simulink model "simulateFlight"  (R2024b)
settings: Solver=VariableStepAuto  StartTime=0.0  StopTime=10
undefined symbols (not defined in the file): aerodynamicData, aircraftConfiguration, alpha0, inertialData, propulsionData, q0, theta0, V0, xE0, zE0
libraries: simulink_extras x8, aerolibatmos2 x2, aerolibanim x1, simulink x1
settings Model: NumberOfSteps=10  VariantFading=off  Creator=vince  LastModifiedBy=klakhara
settings SolverCC: ZeroCrossAlgorithm=Adaptive
settings DebuggingCC: AlgebraicLoopMsg=none  IgnoredZcDiagnostic=none
settings RTWCC: GPUComputeCapability=3.5

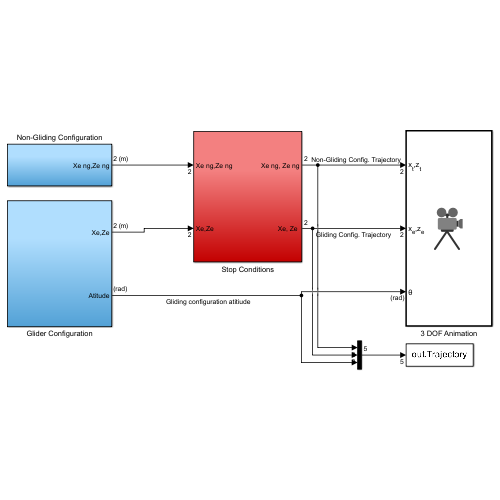
[thumbnail: Simulink's stored preview of the top-level diagram]
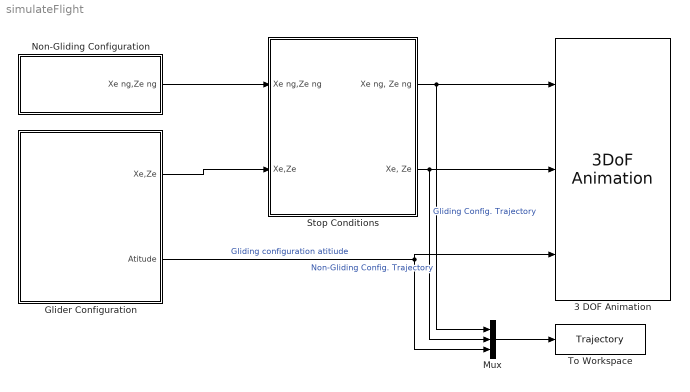
== system simulateFlight ==
  3 DOF Animation : aerolibanim/3DoF Animation  u1=[0 100 0 100 -100 0]  u2=0.01  u3=0.15  u5=Fixed position  u6=[0 50 -0]  u7=40  u8=on
  Glider Configuration : Subsystem
  Mux : Mux  Inputs=3
  Non-Gliding Configuration : Subsystem
  Stop Conditions : Subsystem
  To Workspace : ToWorkspace  VariableName=Trajectory  SaveFormat=Timeseries  SampleTime=-1
  wires:
  Non-Gliding Configuration/1(Xe ng,Ze ng) -> Stop Conditions/1(Xe ng,Ze ng)
  Stop Conditions/1("Xe ng, Ze ng") -> Mux/1, 3 DOF Animation/1  "Non-Gliding Config. Trajectory"
  Glider Configuration/2(Atitude) -> 3 DOF Animation/3, Mux/3  "Gliding configuration atitiude"
  Glider Configuration/1(Xe,Ze) -> Stop Conditions/2(Xe,Ze)
  Stop Conditions/2("Xe, Ze ") -> Mux/2, 3 DOF Animation/2  "Gliding Config. Trajectory"
  Mux/1 -> To Workspace/1

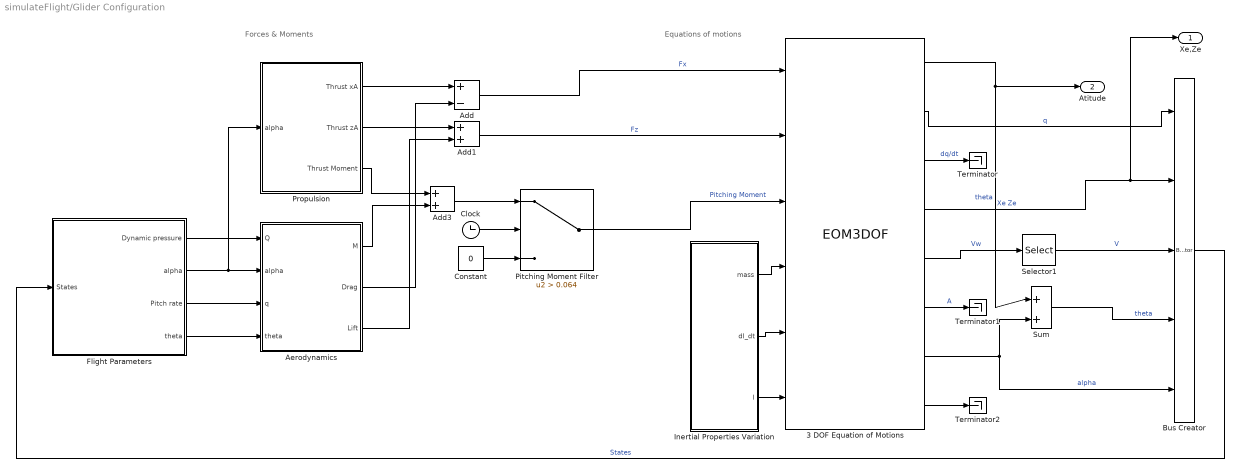
== system simulateFlight/Glider Configuration ==
  note: Forces & Moments
  note: Equations of motions
  3 DOF Equation of Motions : EOM3DOF  axes=Wind  mtype=Custom Variable  v_ini=V0  theta_ini=theta0  gamma_ini=theta0-alpha0  q_ini=q0  alpha_ini=alpha0  pos_ini=[xE0 -zE0]  mass=1  Iyy=1  abi_flag=on
  Add : Sum  Inputs=+-
  Add1 : Sum
  Add3 : Sum
  Aerodynamics : Subsystem
  Bus Creator : BusCreator  Inputs=5
  Clock : Clock
  Constant : Constant  Value=0
  Flight Parameters : Subsystem
  Inertial Properties Variation : Subsystem
  Pitching Moment Filter : Switch  Criteria=u2 > Threshold  Threshold=0.064  SaturateOnIntegerOverflow=off  InputSameDT=off
  Propulsion : Subsystem
  Selector1 : Selector  InputPortWidth=2  IndexOptions=Index vector (dialog)  Indices=[1]  OutputSizes=1
  Sum : Sum  Inputs=|++
  Terminator : Terminator
  Terminator1 : Terminator
  Terminator2 : Terminator
  Xe,Ze : Outport  InitialOutput=0  VectorParamsAs1DForOutWhenUnconnected=off
  Atitude : Outport  Port=2
  wires:
  3 DOF Equation of Motions/5 -> Selector1/1  "Vw"
  Inertial Properties Variation/3(I) -> 3 DOF Equation of Motions/6
  3 DOF Equation of Motions/2 -> Bus Creator/1  "q"
  Pitching Moment Filter/1 -> 3 DOF Equation of Motions/3  "Pitching Moment"
  Inertial Properties Variation/1(mass) -> 3 DOF Equation of Motions/4
  Inertial Properties Variation/2(dI_dt) -> 3 DOF Equation of Motions/5
  3 DOF Equation of Motions/3 -> Terminator/1  "dq/dt"
  3 DOF Equation of Motions/6 -> Terminator1/1  "A"
  Propulsion/3(Thrust Moment) -> Add3/1
  Aerodynamics/1(" M") -> Add3/2
  Aerodynamics/3(Lift) -> Add1/2
  Propulsion/1(Thrust xA) -> Add/1
  Propulsion/2(Thrust zA) -> Add1/1
  Aerodynamics/2(Drag) -> Add/2
  Add1/1 -> 3 DOF Equation of Motions/2  "Fz"
  Add/1 -> 3 DOF Equation of Motions/1  "Fx"
  Add3/1 -> Pitching Moment Filter/1
  3 DOF Equation of Motions/8 -> Terminator2/1
  3 DOF Equation of Motions/7 -> Sum/2, Bus Creator/5  "alpha"
  Selector1/1 -> Bus Creator/3  "V"
  3 DOF Equation of Motions/4 -> Xe,Ze/1, Bus Creator/2  "Xe Ze"
  3 DOF Equation of Motions/1 -> Sum/1, Atitude/1  "theta"
  Flight Parameters/2(alpha) -> Propulsion/1(alpha), Aerodynamics/2(alpha)
  Bus Creator/1 -> Flight Parameters/1(States)  "States"
  Clock/1 -> Pitching Moment Filter/2
  Constant/1 -> Pitching Moment Filter/3
  Flight Parameters/3(Pitch rate) -> Aerodynamics/3(q)
  Flight Parameters/4(theta) -> Aerodynamics/4(theta)
  Flight Parameters/1(Dynamic pressure) -> Aerodynamics/1(Q)
  Sum/1 -> Bus Creator/4  "theta"

== system simulateFlight/Non-Gliding Configuration ==
  Aerodynamics & Equations of Motion : Subsystem
  Dynamic pressure Computation : Subsystem
  Hold : Subsystem
  Thrust Profile : Subsystem
  Xe ng,Ze ng : Outport  InitialOutput=0  VectorParamsAs1DForOutWhenUnconnected=off
  wires:
  Dynamic pressure Computation/1(Q) -> Aerodynamics & Equations of Motion/1(Q)
  Aerodynamics & Equations of Motion/5(Attitude) -> Hold/5(theta)
  Thrust Profile/1(Thrust) -> Aerodynamics & Equations of Motion/5(Thrust)
  Aerodynamics & Equations of Motion/1(V(wind)) -> Hold/1("V(wind) ")
  Aerodynamics & Equations of Motion/2(alpha new) -> Hold/2(alpha)
  Aerodynamics & Equations of Motion/3(q new) -> Hold/3("q ")
  Hold/4(q hold) -> Aerodynamics & Equations of Motion/3(q)
  Hold/1(Xe,Ze hold) -> Dynamic pressure Computation/1("Xe, Ze")
  Hold/2(V(wind) hold) -> Dynamic pressure Computation/2(V(wind))
  Hold/3(alpha hold) -> Aerodynamics & Equations of Motion/2(alpha)
  Hold/5(theta hold) -> Aerodynamics & Equations of Motion/4(theta)
  Aerodynamics & Equations of Motion/4(Xe,Ze) -> Hold/4(Xe,Ze), Xe ng,Ze ng/1

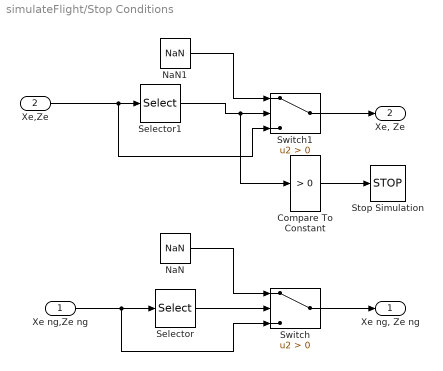
== system simulateFlight/Stop Conditions ==
  Xe ng,Ze ng : Inport
  Xe,Ze : Inport  Port=2
  Compare To Constant : simulink/Logic and Bit Operations/Compare To Constant  relop=>  const=0  OutDataTypeStr=boolean
  NaN : Constant  Value=NaN  OutDataTypeStr=Inherit: Inherit via back propagation
  NaN1 : Constant  Value=NaN  OutDataTypeStr=Inherit: Inherit via back propagation
  Selector : Selector  InputPortWidth=2  IndexOptions=Index vector (dialog)  Indices=[2]  OutputSizes=1
  Selector1 : Selector  InputPortWidth=2  IndexOptions=Index vector (dialog)  Indices=[2]  OutputSizes=1
  Stop Simulation : Stop
  Switch : Switch  Criteria=u2 > Threshold  SaturateOnIntegerOverflow=off  InputSameDT=off
  Switch1 : Switch  Criteria=u2 > Threshold  SaturateOnIntegerOverflow=off  InputSameDT=off
  "Xe ng, Ze ng" : Outport
  "Xe, Ze " : Outport  Port=2
  wires:
  Compare To Constant/1 -> Stop Simulation/1
  Selector/1 -> Switch/2
  NaN/1 -> Switch/1
  Switch/1 -> "Xe ng, Ze ng"/1
  Xe ng,Ze ng/1 -> Switch/3, Selector/1
  Xe,Ze/1 -> Switch1/3, Selector1/1
  Selector1/1 -> Compare To Constant/1, Switch1/2
  NaN1/1 -> Switch1/1
  Switch1/1 -> "Xe, Ze "/1

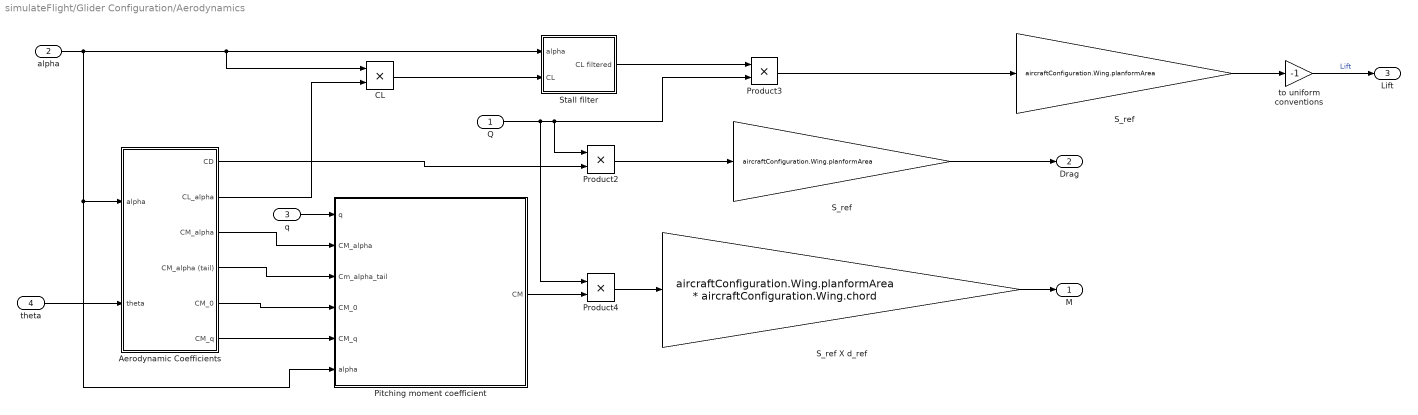
== system simulateFlight/Glider Configuration/Aerodynamics ==
  Q : Inport
  alpha : Inport  Port=2
  q : Inport  Port=3
  theta : Inport  Port=4
  Aerodynamic Coefficients : Subsystem
  CL : Product
  Pitching moment coefficient : Subsystem
  Product2 : Product  InputSameDT=on  SaturateOnIntegerOverflow=on  OutDataTypeStr=Inherit: Same as first input
  Product3 : Product  InputSameDT=on  SaturateOnIntegerOverflow=on  OutDataTypeStr=Inherit: Same as first input
  Product4 : Product  InputSameDT=on  SaturateOnIntegerOverflow=on  OutDataTypeStr=Inherit: Same as first input
  S_ref : Gain  Gain=aircraftConfiguration.Wing.planformArea  SaturateOnIntegerOverflow=on  OutDataTypeStr=Inherit: Same as input  ParamDataTypeStr=Inherit: Same as input
  "S_ref " : Gain  Gain=aircraftConfiguration.Wing.planformArea  SaturateOnIntegerOverflow=on  OutDataTypeStr=Inherit: Same as input  ParamDataTypeStr=Inherit: Same as input
  S_ref X d_ref : Gain  Gain=aircraftConfiguration.Wing.planformArea * aircraftConfiguration.Wing.chord  SaturateOnIntegerOverflow=on  OutDataTypeStr=Inherit: Same as input  ParamDataTypeStr=Inherit: Same as input
  Stall filter : Subsystem
  to uniform conventions : Gain  Gain=-1
  " M" : Outport  InitialOutput=0  VectorParamsAs1DForOutWhenUnconnected=off
  Drag : Outport  Port=2  InitialOutput=[0]  VectorParamsAs1DForOutWhenUnconnected=off
  Lift : Outport  Port=3  InitialOutput=0  VectorParamsAs1DForOutWhenUnconnected=off
  wires:
  theta/1 -> Aerodynamic Coefficients/2(theta)
  alpha/1 -> Stall filter/1(alpha), CL/1, Pitching moment coefficient/6(alpha), Aerodynamic Coefficients/1(alpha)
  S_ref X d_ref/1 -> " M"/1
  q/1 -> Pitching moment coefficient/1(q)
  Aerodynamic Coefficients/2(CL_alpha) -> CL/2
  Aerodynamic Coefficients/1(CD) -> Product2/2
  Aerodynamic Coefficients/3(CM_alpha) -> Pitching moment coefficient/2(CM_alpha)
  Aerodynamic Coefficients/4(CM_alpha (tail)) -> Pitching moment coefficient/3(Cm_alpha_tail)
  Aerodynamic Coefficients/5(CM_0) -> Pitching moment coefficient/4(CM_0)
  Aerodynamic Coefficients/6(CM_q) -> Pitching moment coefficient/5(CM_q)
  CL/1 -> Stall filter/2(CL)
  Q/1 -> Product3/2, Product2/1, Product4/1
  "S_ref "/1 -> to uniform conventions/1
  Pitching moment coefficient/1(CM) -> Product4/2
  Stall filter/1(CL filtered) -> Product3/1
  Product2/1 -> S_ref/1
  Product4/1 -> S_ref X d_ref/1
  Product3/1 -> "S_ref "/1
  S_ref/1 -> Drag/1
  to uniform conventions/1 -> Lift/1  "Lift"

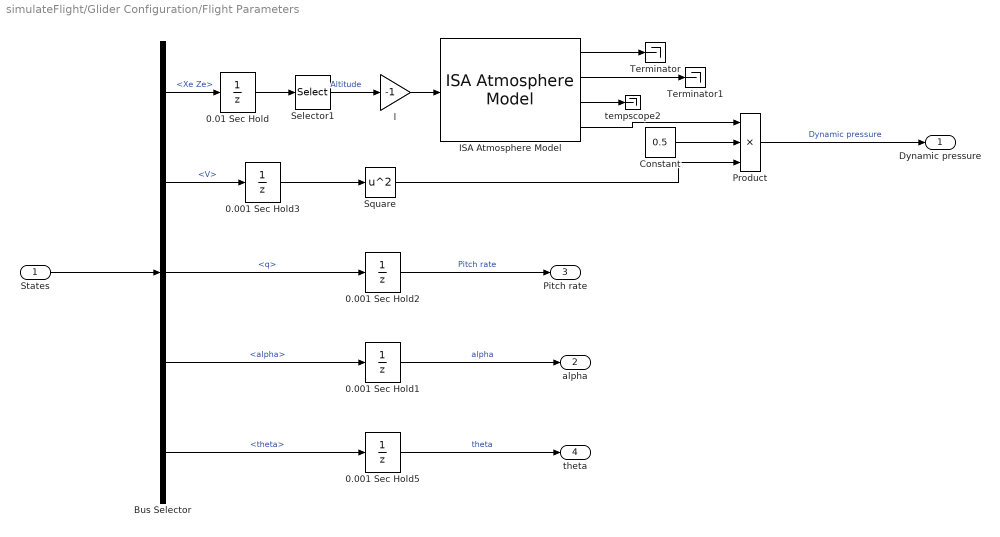
== system simulateFlight/Glider Configuration/Flight Parameters ==
  States : Inport
  0.001 Sec Hold1 : UnitDelay  InitialCondition=alpha0  SampleTime=0.001  HasFrameUpgradeWarning=on
  0.001 Sec Hold2 : UnitDelay  InitialCondition=q0  SampleTime=0.001  HasFrameUpgradeWarning=on
  0.001 Sec Hold3 : UnitDelay  InitialCondition=V0  SampleTime=0.001  HasFrameUpgradeWarning=on
  0.001 Sec Hold5 : UnitDelay  InitialCondition=theta0  SampleTime=0.001  HasFrameUpgradeWarning=on
  0.01 Sec Hold : UnitDelay  InitialCondition=[xE0 -zE0]  SampleTime=0.01  HasFrameUpgradeWarning=on
  Bus Selector : BusSelector  OutputSignals=Xe Ze,V,q,alpha,theta
  Constant : Constant  Value=0.5
  ISA Atmosphere Model : aerolibatmos2/ISA Atmosphere Model  useExtended=off  action=Warning  custom=off  viscosityOut=off  g=9.80665  gamma=1.4  R=287.0531  L=0.0065  h_trop=11000  h_strat=20000  rho0=1.225  P0=101325  T0=288.15  h0=0  S=110.4  Tref=273.15  muref=1.716e-5
  Product : Product  Inputs=3
  Selector1 : Selector  InputPortWidth=2  IndexOptions=Index vector (dialog)  Indices=[2]  OutputSizes=1
  Square : Math  Operator=square
  Terminator : Terminator
  Terminator1 : Terminator
  l : Gain  Gain=-1  SaturateOnIntegerOverflow=on  OutDataTypeStr=Inherit: Same as input  ParamDataTypeStr=Inherit: Same as input
  tempscope2 : Terminator
  Dynamic pressure : Outport
  alpha : Outport  Port=2
  Pitch rate : Outport  Port=3
  theta : Outport  Port=4
  wires:
  Bus Selector/3 -> 0.001 Sec Hold2/1  "<q>"
  Bus Selector/1 -> 0.01 Sec Hold/1  "<Xe Ze>"
  ISA Atmosphere Model/2 -> Terminator1/1
  ISA Atmosphere Model/4 -> Product/1
  0.001 Sec Hold3/1 -> Square/1
  ISA Atmosphere Model/3 -> tempscope2/1
  Bus Selector/2 -> 0.001 Sec Hold3/1  "<V>"
  Bus Selector/4 -> 0.001 Sec Hold1/1  "<alpha>"
  l/1 -> ISA Atmosphere Model/1
  0.001 Sec Hold2/1 -> Pitch rate/1  "Pitch rate"
  Selector1/1 -> l/1  "Altitude"
  0.01 Sec Hold/1 -> Selector1/1
  Bus Selector/5 -> 0.001 Sec Hold5/1  "<theta>"
  Square/1 -> Product/3
  Product/1 -> Dynamic pressure/1  "Dynamic pressure"
  ISA Atmosphere Model/1 -> Terminator/1
  States/1 -> Bus Selector/1
  0.001 Sec Hold5/1 -> theta/1  "theta"
  0.001 Sec Hold1/1 -> alpha/1  "alpha"
  Constant/1 -> Product/2

== system simulateFlight/Glider Configuration/Inertial Properties Variation ==
  Clock : Clock
  Derivative : Derivative
  Inertia moment vs time : Lookup_n-D  NumberOfTableDimensions=1  BreakpointsForDimension1=inertialData.massTimeRange  Table=inertialData.inertiaVector  InternalRulePriority=Speed  RndMeth=Simplest
  mass vs time : Lookup_n-D  NumberOfTableDimensions=1  BreakpointsForDimension1=inertialData.massTimeRange  Table=inertialData.massVector  ExtrapMethod=Clip  InternalRulePriority=Speed  RndMeth=Simplest
  mass : Outport
  dI_dt : Outport  Port=2
  I : Outport  Port=3
  wires:
  Clock/1 -> mass vs time/1, Inertia moment vs time/1
  mass vs time/1 -> mass/1
  Derivative/1 -> dI_dt/1
  Inertia moment vs time/1 -> I/1, Derivative/1

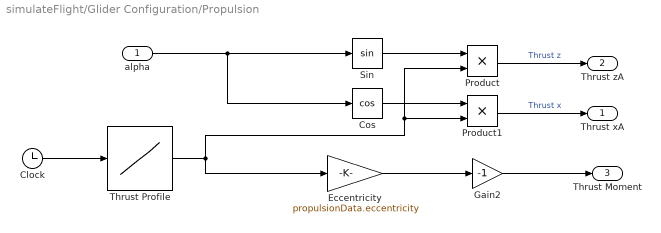
== system simulateFlight/Glider Configuration/Propulsion ==
  alpha : Inport
  Clock : Clock
  Cos : Trigonometry  Operator=cos
  Eccentricity : Gain  Gain=propulsionData.eccentricity
  Gain2 : Gain  Gain=-1
  Product : Product
  Product1 : Product
  Sin : Trigonometry
  Thrust Profile : Lookup_n-D  NumberOfTableDimensions=1  BreakpointsForDimension1=propulsionData.thrustTimeRange  Table=propulsionData.thrustVector  InternalRulePriority=Speed  RndMeth=Simplest
  Thrust xA : Outport
  Thrust zA : Outport  Port=2
  Thrust Moment : Outport  Port=3
  wires:
  alpha/1 -> Cos/1, Sin/1
  Cos/1 -> Product1/1
  Sin/1 -> Product/1
  Product/1 -> Thrust zA/1  "Thrust z"
  Product1/1 -> Thrust xA/1  "Thrust x"
  Thrust Profile/1 -> Eccentricity/1, Product1/2, Product/2
  Eccentricity/1 -> Gain2/1
  Gain2/1 -> Thrust Moment/1
  Clock/1 -> Thrust Profile/1

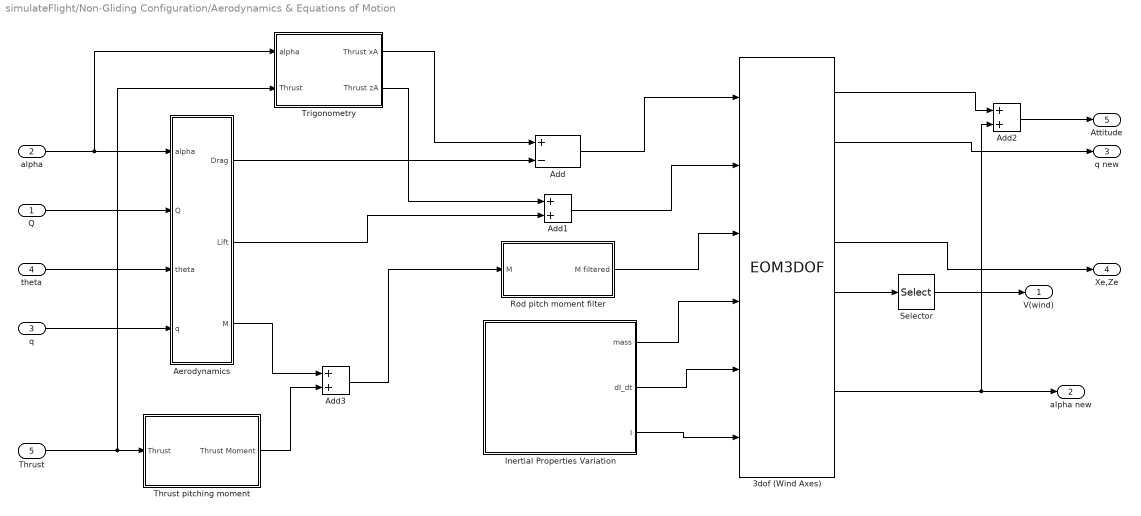
== system simulateFlight/Non-Gliding Configuration/Aerodynamics & Equations of Motion ==
  Q : Inport
  alpha : Inport  Port=2
  q : Inport  Port=3
  theta : Inport  Port=4
  Thrust : Inport  Port=5
  3dof (Wind Axes) : EOM3DOF  axes=Wind  mtype=Custom Variable  v_ini=V0  theta_ini=theta0  gamma_ini=theta0-alpha0  q_ini=q0  alpha_ini=alpha0  pos_ini=[xE0 zE0]  abi_flag=on
  Add : Sum  Inputs=+-
  Add1 : Sum
  Add2 : Sum
  Add3 : Sum
  Aerodynamics : Subsystem
  Inertial Properties Variation : Subsystem
  Rod pitch moment filter : Subsystem
  Selector : Selector  NumberOfDimensions=2  InputPortWidth=3  IndexOptions=Index vector (dialog),Index vector (dialog)  Indices=1,1  OutputSizes=1,1
  Thrust pitching moment : Subsystem
  Trigonometry : Subsystem
  V(wind) : Outport  InitialOutput=0  VectorParamsAs1DForOutWhenUnconnected=off
  alpha new : Outport  Port=2  InitialOutput=0  VectorParamsAs1DForOutWhenUnconnected=off
  q new : Outport  Port=3  InitialOutput=0  VectorParamsAs1DForOutWhenUnconnected=off
  Xe,Ze : Outport  Port=4  InitialOutput=0  VectorParamsAs1DForOutWhenUnconnected=off
  Attitude : Outport  Port=5  InitialOutput=0  VectorParamsAs1DForOutWhenUnconnected=off
  wires:
  Add/1 -> 3dof (Wind Axes)/1
  Q/1 -> Aerodynamics/2(Q)
  3dof (Wind Axes)/4 -> Xe,Ze/1
  3dof (Wind Axes)/1 -> Add2/1
  theta/1 -> Aerodynamics/3(theta)
  alpha/1 -> Aerodynamics/1(alpha), Trigonometry/1(alpha)
  Trigonometry/2(Thrust zA) -> Add1/1
  Aerodynamics/2(Lift) -> Add1/2
  3dof (Wind Axes)/5 -> Selector/1
  Thrust/1 -> Trigonometry/2(Thrust), Thrust pitching moment/1(Thrust)
  3dof (Wind Axes)/2 -> q new/1
  q/1 -> Aerodynamics/4(q)
  Aerodynamics/1(Drag) -> Add/2
  Trigonometry/1(Thrust xA) -> Add/1
  Add1/1 -> 3dof (Wind Axes)/2
  Rod pitch moment filter/1(M filtered) -> 3dof (Wind Axes)/3
  Thrust pitching moment/1(Thrust Moment) -> Add3/2
  Aerodynamics/3(" M") -> Add3/1
  Add3/1 -> Rod pitch moment filter/1(M)
  Inertial Properties Variation/1(mass) -> 3dof (Wind Axes)/4
  Inertial Properties Variation/2(dI_dt) -> 3dof (Wind Axes)/5
  Inertial Properties Variation/3(I) -> 3dof (Wind Axes)/6
  Selector/1 -> V(wind)/1
  3dof (Wind Axes)/7 -> Add2/2, alpha new/1
  Add2/1 -> Attitude/1

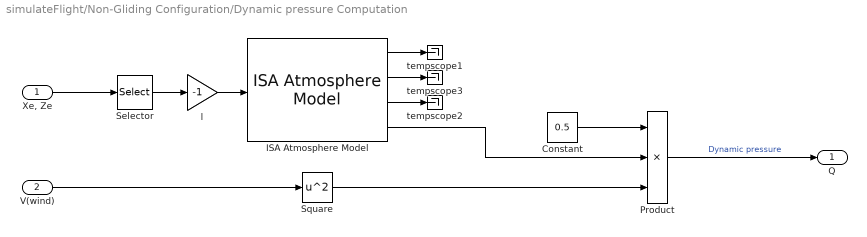
== system simulateFlight/Non-Gliding Configuration/Dynamic pressure Computation ==
  "Xe, Ze" : Inport
  V(wind) : Inport  Port=2
  Constant : Constant  Value=0.5
  ISA Atmosphere Model : aerolibatmos2/ISA Atmosphere Model  useExtended=off  action=Warning  custom=off  viscosityOut=off  g=9.80665  gamma=1.4  R=287.0531  L=0.0065  h_trop=11000  h_strat=20000  rho0=1.225  P0=101325  T0=288.15  h0=0  S=110.4  Tref=273.15  muref=1.716e-5
  Product : Product  Inputs=3
  Selector : Selector  InputPortWidth=2  IndexOptions=Index vector (dialog)  Indices=[2]  OutputSizes=1
  Square : Math  Operator=square
  l : Gain  Gain=-1  SaturateOnIntegerOverflow=on  OutDataTypeStr=Inherit: Same as input  ParamDataTypeStr=Inherit: Same as input
  tempscope1 : Terminator
  tempscope2 : Terminator
  tempscope3 : Terminator
  Q : Outport
  wires:
  l/1 -> ISA Atmosphere Model/1
  ISA Atmosphere Model/1 -> tempscope1/1
  ISA Atmosphere Model/3 -> tempscope2/1
  Selector/1 -> l/1
  Product/1 -> Q/1  "Dynamic pressure"
  Constant/1 -> Product/1
  ISA Atmosphere Model/4 -> Product/2
  Square/1 -> Product/3
  "Xe, Ze"/1 -> Selector/1
  V(wind)/1 -> Square/1
  ISA Atmosphere Model/2 -> tempscope3/1

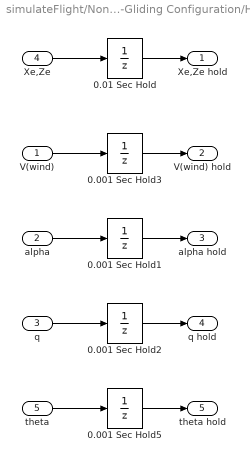
== system simulateFlight/Non-Gliding Configuration/Hold ==
  "V(wind) " : Inport
  alpha : Inport  Port=2
  "q " : Inport  Port=3
  Xe,Ze : Inport  Port=4
  theta : Inport  Port=5
  0.001 Sec Hold1 : UnitDelay  InitialCondition=alpha0  SampleTime=0.001  HasFrameUpgradeWarning=on
  0.001 Sec Hold2 : UnitDelay  InitialCondition=q0  SampleTime=0.001  HasFrameUpgradeWarning=on
  0.001 Sec Hold3 : UnitDelay  InitialCondition=V0  SampleTime=0.001  HasFrameUpgradeWarning=on
  0.001 Sec Hold5 : UnitDelay  InitialCondition=theta0  SampleTime=0.001  HasFrameUpgradeWarning=on
  0.01 Sec Hold : UnitDelay  InitialCondition=[xE0 -zE0]  SampleTime=0.01  HasFrameUpgradeWarning=on
  Xe,Ze hold : Outport
  V(wind) hold : Outport  Port=2
  alpha hold : Outport  Port=3
  q hold : Outport  Port=4
  theta hold : Outport  Port=5
  wires:
  alpha/1 -> 0.001 Sec Hold1/1
  0.001 Sec Hold3/1 -> V(wind) hold/1
  "V(wind) "/1 -> 0.001 Sec Hold3/1
  Xe,Ze/1 -> 0.01 Sec Hold/1
  "q "/1 -> 0.001 Sec Hold2/1
  0.001 Sec Hold2/1 -> q hold/1
  0.01 Sec Hold/1 -> Xe,Ze hold/1
  0.001 Sec Hold1/1 -> alpha hold/1
  theta/1 -> 0.001 Sec Hold5/1
  0.001 Sec Hold5/1 -> theta hold/1

== system simulateFlight/Non-Gliding Configuration/Thrust Profile ==
  1-D Lookup Table : Lookup_n-D  NumberOfTableDimensions=1  BreakpointsForDimension1=propulsionData.thrustTimeRange  Table=propulsionData.thrustVector  InternalRulePriority=Speed  RndMeth=Simplest
  Clock : Clock
  Scope : Scope  NumInputPorts=2
  Thrust : Outport
  wires:
  Clock/1 -> 1-D Lookup Table/1
  1-D Lookup Table/1 -> Scope/1, Thrust/1

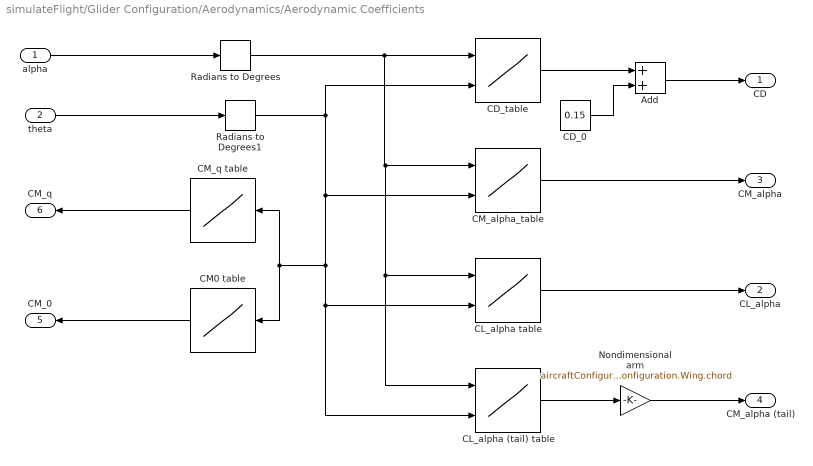
== system simulateFlight/Glider Configuration/Aerodynamics/Aerodynamic Coefficients ==
  alpha : Inport
  theta : Inport  Port=2
  Add : Sum
  CD_0 : Constant  Value=0.15
  CD_table : Lookup_n-D  BreakpointsForDimension1=aerodynamicData.alphaRange  BreakpointsForDimension2=aerodynamicData.thetaRange  Table=aerodynamicData.dragCoefficient.CD_table  ExtrapMethod=Clip  InternalRulePriority=Speed  RndMeth=Simplest
      settings: InputPortMap=u0,u1
  CL_alpha (tail) table : Lookup_n-D  BreakpointsForDimension1=aerodynamicData.alphaRange  BreakpointsForDimension2=aerodynamicData.thetaRange  Table=aerodynamicData.liftCoefficient.CL_alpha_tail_table  InternalRulePriority=Speed  RndMeth=Simplest
      settings: InputPortMap=u0,u1
  CL_alpha table : Lookup_n-D  BreakpointsForDimension1=aerodynamicData.alphaRange  BreakpointsForDimension2=aerodynamicData.thetaRange  Table=aerodynamicData.liftCoefficient.CL_alpha_table  ExtrapMethod=Clip  InternalRulePriority=Speed  RndMeth=Simplest
      settings: InputPortMap=u0,u1
  CM0 table : Lookup_n-D  NumberOfTableDimensions=1  BreakpointsForDimension1=aerodynamicData.thetaRange  Table=aerodynamicData.pitchMomentCoefficient.CM_0  InternalRulePriority=Speed  RndMeth=Simplest
  CM_alpha_table : Lookup_n-D  BreakpointsForDimension1=aerodynamicData.alphaRange  BreakpointsForDimension2=aerodynamicData.thetaRange  Table=aerodynamicData.pitchMomentCoefficient.CM_alpha_table  ExtrapMethod=Clip  InternalRulePriority=Speed  RndMeth=Simplest
      settings: InputPortMap=u0,u1
  CM_q table : Lookup_n-D  NumberOfTableDimensions=1  BreakpointsForDimension1=aerodynamicData.thetaRange  Table=aerodynamicData.pitchMomentCoefficient.Cm_q  InternalRulePriority=Speed  RndMeth=Simplest
  Nondimensional arm : Gain  Gain=aircraftConfiguration.HT.Arm/aircraftConfiguration.Wing.chord
  Radians to Degrees : simulink_extras/Transformations/Radians to Degrees
  Radians to Degrees1 : simulink_extras/Transformations/Radians to Degrees
  CD : Outport
  CL_alpha : Outport  Port=2
  CM_alpha : Outport  Port=3
  CM_alpha (tail) : Outport  Port=4
  CM_0 : Outport  Port=5
  CM_q : Outport  Port=6
  wires:
  alpha/1 -> Radians to Degrees/1
  Radians to Degrees/1 -> CL_alpha (tail) table/1, CL_alpha table/1, CM_alpha_table/1, CD_table/1
  Radians to Degrees1/1 -> CL_alpha (tail) table/2, CL_alpha table/2, CM0 table/1, CM_q table/1, CM_alpha_table/2, CD_table/2
  theta/1 -> Radians to Degrees1/1
  CM_alpha_table/1 -> CM_alpha/1
  CM0 table/1 -> CM_0/1
  Add/1 -> CD/1
  Nondimensional arm/1 -> CM_alpha (tail)/1
  CM_q table/1 -> CM_q/1
  CL_alpha table/1 -> CL_alpha/1
  CL_alpha (tail) table/1 -> Nondimensional arm/1
  CD_table/1 -> Add/1
  CD_0/1 -> Add/2

== system simulateFlight/Glider Configuration/Aerodynamics/Pitching moment coefficient ==
  q : Inport
  CM_alpha : Inport  Port=2
  Cm_alpha_tail : Inport  Port=3
  CM_0 : Inport  Port=4
  CM_q : Inport  Port=5
  alpha : Inport  Port=6
  Add : Sum  Inputs=++++
  CM(a) : Product
  CM(q) : Product
  CM(tail) : Product
  CM_scope : Scope  NumInputPorts=5
  CM : Outport
  wires:
  CM(q)/1 -> Add/4, CM_scope/5
  CM(a)/1 -> Add/2, CM_scope/3
  alpha/1 -> CM(a)/2, CM(tail)/1
  q/1 -> CM(q)/2
  CM(tail)/1 -> Add/3, CM_scope/4
  Add/1 -> CM_scope/1, CM/1  "Resultant"
  CM_q/1 -> CM(q)/1
  CM_alpha/1 -> CM(a)/1
  Cm_alpha_tail/1 -> CM(tail)/2
  CM_0/1 -> Add/1, CM_scope/2

== system simulateFlight/Glider Configuration/Aerodynamics/Stall filter ==
  note: The aircraft stalls at 17 degrees of angle of attack
  alpha : Inport
  CL : Inport  Port=2
  Constant : Constant  Value=0
  Radians to Degrees : simulink_extras/Transformations/Radians to Degrees
  Switch : Switch  Criteria=u2 > Threshold  Threshold=17  SaturateOnIntegerOverflow=off  InputSameDT=off
  CL filtered : Outport
  wires:
  alpha/1 -> Radians to Degrees/1
  Radians to Degrees/1 -> Switch/2
  CL/1 -> Switch/3
  Constant/1 -> Switch/1
  Switch/1 -> CL filtered/1

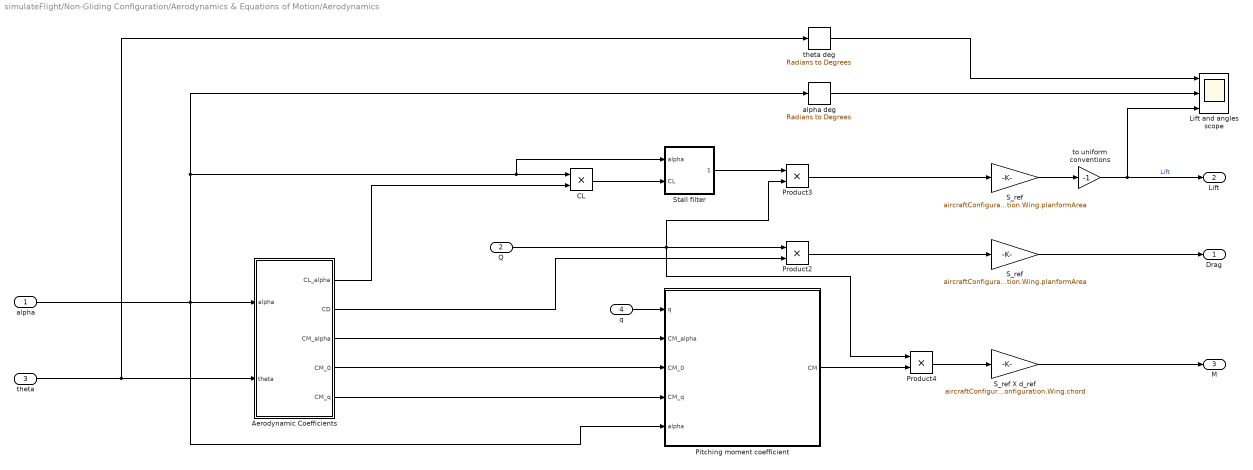
== system simulateFlight/Non-Gliding Configuration/Aerodynamics & Equations of Motion/Aerodynamics ==
  alpha : Inport
  Q : Inport  Port=2
  theta : Inport  Port=3
  q : Inport  Port=4
  Aerodynamic Coefficients : Subsystem
  CL : Product
  Lift and angles scope : Scope  NumInputPorts=3
  Pitching moment coefficient : Subsystem
  Product2 : Product  InputSameDT=on  SaturateOnIntegerOverflow=on  OutDataTypeStr=Inherit: Same as first input
  Product3 : Product  InputSameDT=on  SaturateOnIntegerOverflow=on  OutDataTypeStr=Inherit: Same as first input
  Product4 : Product  InputSameDT=on  SaturateOnIntegerOverflow=on  OutDataTypeStr=Inherit: Same as first input
  S_ref : Gain  Gain=aircraftConfiguration.Wing.planformArea  SaturateOnIntegerOverflow=on  OutDataTypeStr=Inherit: Same as input  ParamDataTypeStr=Inherit: Same as input
  "S_ref " : Gain  Gain=aircraftConfiguration.Wing.planformArea  SaturateOnIntegerOverflow=on  OutDataTypeStr=Inherit: Same as input  ParamDataTypeStr=Inherit: Same as input
  S_ref X d_ref : Gain  Gain=aircraftConfiguration.Wing.planformArea * aircraftConfiguration.Wing.chord  SaturateOnIntegerOverflow=on  OutDataTypeStr=Inherit: Same as input  ParamDataTypeStr=Inherit: Same as input
  Stall filter : Subsystem
  alpha deg : simulink_extras/Transformations/Radians to Degrees
  theta deg : simulink_extras/Transformations/Radians to Degrees
  to uniform conventions : Gain  Gain=-1
  Drag : Outport  InitialOutput=[0]  VectorParamsAs1DForOutWhenUnconnected=off
  Lift : Outport  Port=2  InitialOutput=0  VectorParamsAs1DForOutWhenUnconnected=off
  " M" : Outport  Port=3  InitialOutput=0  VectorParamsAs1DForOutWhenUnconnected=off
  wires:
  Product2/1 -> S_ref/1
  S_ref/1 -> Drag/1
  Q/1 -> Product3/2, Product2/1, Product4/1
  theta/1 -> Aerodynamic Coefficients/2(theta), theta deg/1
  to uniform conventions/1 -> Lift and angles scope/3, Lift/1  "Lift"
  "S_ref "/1 -> to uniform conventions/1
  S_ref X d_ref/1 -> " M"/1
  CL/1 -> Stall filter/2(CL)
  alpha/1 -> Pitching moment coefficient/5(alpha), Aerodynamic Coefficients/1(alpha), alpha deg/1, Stall filter/1(alpha), CL/1
  Pitching moment coefficient/1(CM) -> Product4/2
  Product4/1 -> S_ref X d_ref/1
  Aerodynamic Coefficients/3(CM_alpha) -> Pitching moment coefficient/2(CM_alpha)
  Aerodynamic Coefficients/5(CM_q) -> Pitching moment coefficient/4(CM_q)
  Aerodynamic Coefficients/4(CM_0) -> Pitching moment coefficient/3(CM_0)
  Aerodynamic Coefficients/1(CL_alpha) -> CL/2
  Stall filter/1(CL filtered) -> Product3/1
  Product3/1 -> "S_ref "/1
  Aerodynamic Coefficients/2(CD) -> Product2/2
  theta deg/1 -> Lift and angles scope/1
  alpha deg/1 -> Lift and angles scope/2
  q/1 -> Pitching moment coefficient/1(q)

== system simulateFlight/Non-Gliding Configuration/Aerodynamics & Equations of Motion/Inertial Properties Variation ==
  Clock : Clock
  Derivative : Derivative
  Inertia moment vs time : Lookup_n-D  NumberOfTableDimensions=1  BreakpointsForDimension1=inertialData.massTimeRange  Table=inertialData.inertiaVector  InternalRulePriority=Speed  RndMeth=Simplest
  mass vs time : Lookup_n-D  NumberOfTableDimensions=1  BreakpointsForDimension1=inertialData.massTimeRange  Table=inertialData.massVector  ExtrapMethod=Clip  InternalRulePriority=Speed  RndMeth=Simplest
  mass : Outport
  dI_dt : Outport  Port=2
  I : Outport  Port=3
  wires:
  Clock/1 -> mass vs time/1, Inertia moment vs time/1
  mass vs time/1 -> mass/1
  Derivative/1 -> dI_dt/1
  Inertia moment vs time/1 -> I/1, Derivative/1

== system simulateFlight/Non-Gliding Configuration/Aerodynamics & Equations of Motion/Rod pitch moment filter ==
  note: filter due to the rod at 0.065s,
      | when it leaves the launch tube
  M : Inport
  Clock : Clock
  Constant : Constant  Value=0
  Switch : Switch  Criteria=u2 > Threshold  Threshold=0.064  SaturateOnIntegerOverflow=off  InputSameDT=off
  M filtered : Outport
  wires:
  Clock/1 -> Switch/2
  Constant/1 -> Switch/3
  Switch/1 -> M filtered/1
  M/1 -> Switch/1

== system simulateFlight/Non-Gliding Configuration/Aerodynamics & Equations of Motion/Thrust pitching moment ==
  note: Thrust makes a pitching moment
      | because of the position of the bottle
  Thrust : Inport
  Eccentricity : Gain  Gain=propulsionData.eccentricity
  Gain2 : Gain  Gain=-1
  Thrust Moment : Outport
  wires:
  Eccentricity/1 -> Gain2/1
  Thrust/1 -> Eccentricity/1
  Gain2/1 -> Thrust Moment/1

== system simulateFlight/Non-Gliding Configuration/Aerodynamics & Equations of Motion/Trigonometry ==
  alpha : Inport
  Thrust : Inport  Port=2
  Cos : Trigonometry  Operator=cos
  Product : Product
  Product1 : Product
  Sin : Trigonometry
  Thrust xA : Outport
  Thrust zA : Outport  Port=2
  wires:
  alpha/1 -> Sin/1, Cos/1
  Thrust/1 -> Product/2, Product1/2
  Cos/1 -> Product1/1
  Sin/1 -> Product/1
  Product/1 -> Thrust zA/1
  Product1/1 -> Thrust xA/1

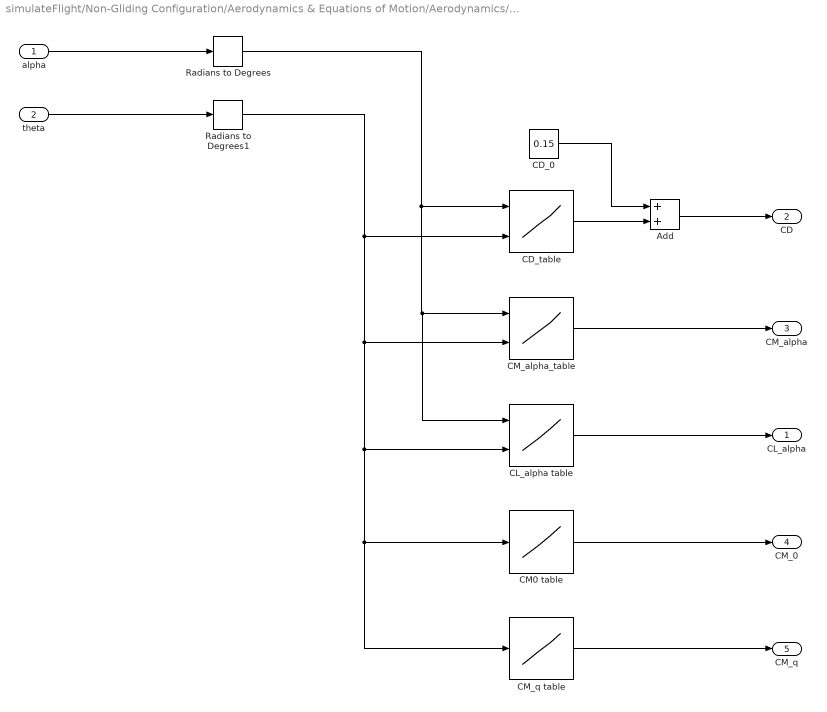
== system simulateFlight/Non-Gliding Configuration/Aerodynamics & Equations of Motion/Aerodynamics/Aerodynamic Coefficients ==
  alpha : Inport
  theta : Inport  Port=2
  Add : Sum
  CD_0 : Constant  Value=0.15
  CD_table : Lookup_n-D  BreakpointsForDimension1=aerodynamicData.alphaRange  BreakpointsForDimension2=aerodynamicData.thetaRange  Table=aerodynamicData.dragCoefficient.CD_table  ExtrapMethod=Clip  InternalRulePriority=Speed  RndMeth=Simplest
      settings: InputPortMap=u0,u1
  CL_alpha table : Lookup_n-D  BreakpointsForDimension1=aerodynamicData.alphaRange  BreakpointsForDimension2=aerodynamicData.thetaRange  Table=aerodynamicData.liftCoefficient.CL_alpha_table  ExtrapMethod=Clip  InternalRulePriority=Speed  RndMeth=Simplest
      settings: InputPortMap=u0,u1
  CM0 table : Lookup_n-D  NumberOfTableDimensions=1  BreakpointsForDimension1=aerodynamicData.thetaRange  Table=aerodynamicData.pitchMomentCoefficient.CM_0  InternalRulePriority=Speed  RndMeth=Simplest
  CM_alpha_table : Lookup_n-D  BreakpointsForDimension1=aerodynamicData.alphaRange  BreakpointsForDimension2=aerodynamicData.thetaRange  Table=aerodynamicData.pitchMomentCoefficient.CM_alpha_table  ExtrapMethod=Clip  InternalRulePriority=Speed  RndMeth=Simplest
      settings: InputPortMap=u0,u1
  CM_q table : Lookup_n-D  NumberOfTableDimensions=1  BreakpointsForDimension1=aerodynamicData.thetaRange  Table=aerodynamicData.pitchMomentCoefficient.Cm_q  InternalRulePriority=Speed  RndMeth=Simplest
  Radians to Degrees : simulink_extras/Transformations/Radians to Degrees
  Radians to Degrees1 : simulink_extras/Transformations/Radians to Degrees
  CL_alpha : Outport
  CD : Outport  Port=2
  CM_alpha : Outport  Port=3
  CM_0 : Outport  Port=4
  CM_q : Outport  Port=5
  wires:
  alpha/1 -> Radians to Degrees/1
  Radians to Degrees/1 -> CL_alpha table/1, CM_alpha_table/1, CD_table/1
  Radians to Degrees1/1 -> CM_q table/1, CM0 table/1, CL_alpha table/2, CM_alpha_table/2, CD_table/2
  theta/1 -> Radians to Degrees1/1
  CM_alpha_table/1 -> CM_alpha/1
  CL_alpha table/1 -> CL_alpha/1
  CM0 table/1 -> CM_0/1
  CD_table/1 -> Add/2
  Add/1 -> CD/1
  CD_0/1 -> Add/1
  CM_q table/1 -> CM_q/1

== system simulateFlight/Non-Gliding Configuration/Aerodynamics & Equations of Motion/Aerodynamics/Pitching moment coefficient ==
  q : Inport
  CM_alpha : Inport  Port=2
  CM_0 : Inport  Port=3
  CM_q : Inport  Port=4
  alpha : Inport  Port=5
  Add : Sum  Inputs=+++
  CM(a) : Product
  CM(q) : Product
  CM_scope : Scope  NumInputPorts=4
  CM : Outport
  wires:
  CM(q)/1 -> CM_scope/4, Add/3
  CM(a)/1 -> Add/2, CM_scope/3
  alpha/1 -> CM(a)/2
  q/1 -> CM(q)/2
  Add/1 -> CM_scope/1, CM/1  "Resultant"
  CM_q/1 -> CM(q)/1
  CM_alpha/1 -> CM(a)/1
  CM_0/1 -> Add/1, CM_scope/2

== system simulateFlight/Non-Gliding Configuration/Aerodynamics & Equations of Motion/Aerodynamics/Stall filter ==
  note: The aircraft stalls at 17 degrees of angle of attack
  alpha : Inport
  CL : Inport  Port=2
  Constant : Constant  Value=0
  Radians to Degrees : simulink_extras/Transformations/Radians to Degrees
  Switch : Switch  Criteria=u2 > Threshold  Threshold=17  SaturateOnIntegerOverflow=off  InputSameDT=off
  CL filtered : Outport
  wires:
  alpha/1 -> Radians to Degrees/1
  Radians to Degrees/1 -> Switch/2
  CL/1 -> Switch/3
  Constant/1 -> Switch/1
  Switch/1 -> CL filtered/1
